simulink model "Atomic_Subsystem"  (R2020a)
settings: Solver=VariableStepAuto  StartTime=0.0  StopTime=10.0  RelTol=1e-3
settings Model: Creator=shweta  LastModifiedBy=shweta
settings DataIOCC: SaveOutput=off  SaveTime=off

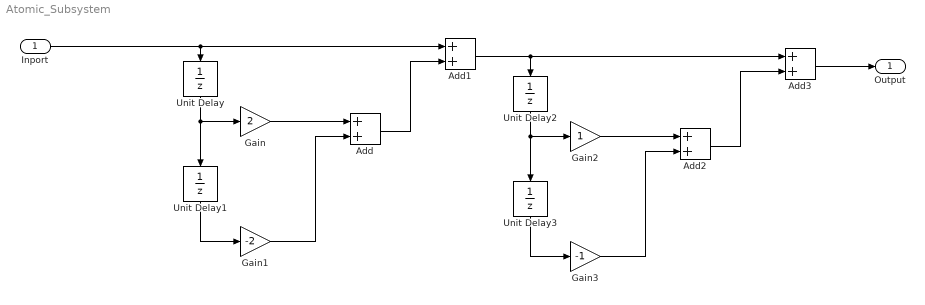
== system Atomic_Subsystem ==
  Inport : Inport  OutDataTypeStr=double  PortDimensions=1  SampleTime=0
  Add{,1..3} (4 alike) : Sum
  Gain : Gain  Gain=2
  Gain1 : Gain  Gain=-2
  Gain2 : Gain
  Gain3 : Gain  Gain=-1
  Unit Delay{,1..3} (4 alike) : UnitDelay  SampleTime=-1  HasFrameUpgradeWarning=on
  Output : Outport  OutDataTypeStr=double  PortDimensions=1  SampleTime=0
  wires:
  Gain3/1 -> Add2/2
  Unit Delay2/1 -> Gain2/1, Unit Delay3/1
  Gain2/1 -> Add2/1
  Add3/1 -> Output/1
  Add2/1 -> Add3/2
  Add1/1 -> Add3/1, Unit Delay2/1
  Add/1 -> Add1/2
  Unit Delay1/1 -> Gain1/1
  Gain/1 -> Add/1
  Unit Delay/1 -> Gain/1, Unit Delay1/1
  Inport/1 -> Unit Delay/1, Add1/1
  Unit Delay3/1 -> Gain3/1
  Gain1/1 -> Add/2
